simulink model "ScenarioNew"  (Simulink 7.7)
settings: Solver=ode45  StartTime=0.0  StopTime=10.0  RelTol=1e-3
undefined symbols (not defined in the file): sigbuilder_block
libraries: simulink x1
settings Model: Creator=Zsolt  LastModifiedBy=jscott
settings HardwareCC: TargetIntDivRoundTo=Zero  TargetEndianess=LittleEndian  TargetHWDeviceType=MATLAB Host  ProdEqTarget=off
settings RTWCC: SystemTargetFile=rsim.tlc  TemplateMakefile=rsim_default_tmf  Description=Rapid Simulation Target  ProcessScript=rsim_make_rtw_hook
settings RSimTargetCC: TargetFunctionLibrary=ANSI_C  ERTMultiwordTypeDef=System defined  FunctionExecutionProfile=off  CodeExecutionProfiling=off  ERTCodeCoverageTool=None  ERTMultiwordLength=256  IsPILTarget=off  EnableShiftOperators=on  PortableWordSizes=off

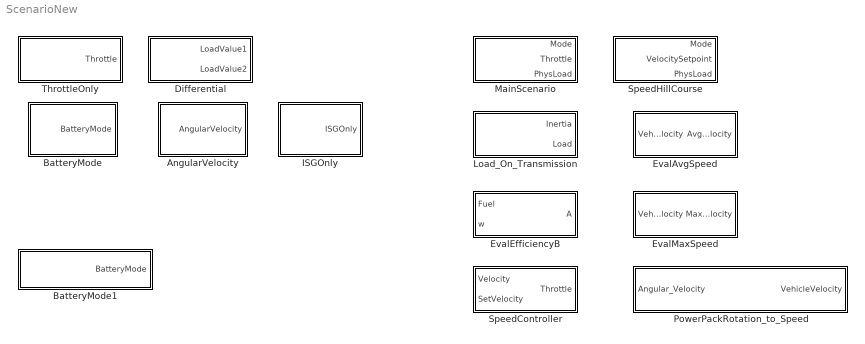
== system ScenarioNew ==
  AngularVelocity : Subsystem  Tag=STV Subsys  LoadFcn=sigbuilder_block('load');  StartFcn=sigbuilder_block('start');  StopFcn=sigbuilder_block('stop');  ClipboardFcn=sigbuilder_block('clipboard');  mask(Sigbuilder block){}
      mask help: Create and generate interchangeable groups of signals whose waveforms are piecewise linear.
      mask init:
      | if ~strcmp(get_param(bdroot(gcbh),'SimulationStatus'),'stopped') tuvar = sigbuilder_block('maskInit'); end
      settings: CopyFcn=sigbuilder_block('copy');  DeleteFcn=sigbuilder_block('delete');  ModelCloseFcn=sigbuilder_block('modelClose');  PreSaveFcn=sigbuilder_block('preSave');  NameChangeFcn=sigbuilder_block('namechange');  OpenFcn=sigbuilder_block('open',[437.25 199.5 550.5 399.75 ]);  CloseFcn=sigbuilder_block('close');
      mask Display: plot(0,0,100,100,[10,10,40,40,10],[80,20,20,80,80],[40,10],[50,50], [40,27,10],[65,72,56],[40,25,25,10],[28,28,43,43]);
  BatteryMode : Subsystem  Tag=STV Subsys  LoadFcn=sigbuilder_block('load');  StartFcn=sigbuilder_block('start');  StopFcn=sigbuilder_block('stop');  ClipboardFcn=sigbuilder_block('clipboard');  mask(Sigbuilder block){}
      mask help: Create and generate interchangeable groups of signals whose waveforms are piecewise linear.
      mask init:
      | if ~strcmp(get_param(bdroot(gcbh),'SimulationStatus'),'stopped') tuvar = sigbuilder_block('maskInit'); end
      settings: CopyFcn=sigbuilder_block('copy');  DeleteFcn=sigbuilder_block('delete');  ModelCloseFcn=sigbuilder_block('modelClose');  PreSaveFcn=sigbuilder_block('preSave');  NameChangeFcn=sigbuilder_block('namechange');  OpenFcn=sigbuilder_block('open',[437.25 199.5 550.5 399.75 ]);  CloseFcn=sigbuilder_block('close');
      mask Display: plot(0,0,100,100,[10,10,40,40,10],[80,20,20,80,80],[40,10],[50,50], [40,27,10],[65,72,56],[40,25,25,10],[28,28,43,43]);
  BatteryMode1 : Subsystem  Tag=STV Subsys  LoadFcn=sigbuilder_block('load');  StartFcn=sigbuilder_block('start');  StopFcn=sigbuilder_block('stop');  ClipboardFcn=sigbuilder_block('clipboard');  mask(Sigbuilder block){}
      mask help: Create and generate interchangeable groups of signals whose waveforms are piecewise linear.
      mask init:
      | if ~strcmp(get_param(bdroot(gcbh),'SimulationStatus'),'stopped') tuvar = sigbuilder_block('maskInit'); end
      settings: CopyFcn=sigbuilder_block('copy');  DeleteFcn=sigbuilder_block('delete');  ModelCloseFcn=sigbuilder_block('modelClose');  PreSaveFcn=sigbuilder_block('preSave');  NameChangeFcn=sigbuilder_block('namechange');  OpenFcn=sigbuilder_block('open',[437.25 199.5 550.5 399.75 ]);  CloseFcn=sigbuilder_block('close');
      mask Display: plot(0,0,100,100,[10,10,40,40,10],[80,20,20,80,80],[40,10],[50,50], [40,27,10],[65,72,56],[40,25,25,10],[28,28,43,43]);
  Differential : Subsystem
  EvalAvgSpeed : Subsystem
  EvalEfficiencyB : Subsystem
  EvalMaxSpeed : Subsystem
  ISGOnly : Subsystem  Tag=STV Subsys  LoadFcn=sigbuilder_block('load');  StartFcn=sigbuilder_block('start');  StopFcn=sigbuilder_block('stop');  ClipboardFcn=sigbuilder_block('clipboard');  mask(Sigbuilder block){}
      mask help: Create and generate interchangeable groups of signals whose waveforms are piecewise linear.
      mask init:
      | if ~strcmp(get_param(bdroot(gcbh),'SimulationStatus'),'stopped') tuvar = sigbuilder_block('maskInit'); end
      settings: CopyFcn=sigbuilder_block('copy');  DeleteFcn=sigbuilder_block('delete');  ModelCloseFcn=sigbuilder_block('modelClose');  PreSaveFcn=sigbuilder_block('preSave');  NameChangeFcn=sigbuilder_block('namechange');  OpenFcn=sigbuilder_block('open',[437.25 199.5 550.5 399.75 ]);  CloseFcn=sigbuilder_block('close');
      mask Display: plot(0,0,100,100,[10,10,40,40,10],[80,20,20,80,80],[40,10],[50,50], [40,27,10],[65,72,56],[40,25,25,10],[28,28,43,43]);
  Load_On_Transmission : Subsystem
  MainScenario : Subsystem
  PowerPackRotation_to_Speed : Subsystem
  SpeedController : Subsystem
  SpeedHillCourse : Subsystem
  ThrottleOnly : Subsystem

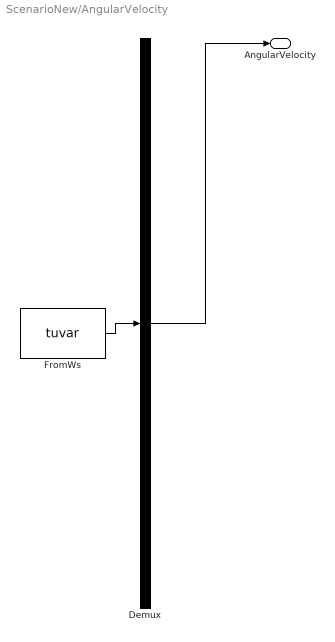
== system ScenarioNew/AngularVelocity ==
  Demux : Demux  Tag=STV Demux  Outputs=1
  FromWs : FromWorkspace  Tag=STV FromWs  VariableName=tuvar  SampleTime=0  SigBuilderData=DataTag0  VnvData=DataTag1
      SigBuilderData=|
      | common.afterFinalStr = 'Extrapolate'
      | common.sampleTime = 0
      | dataSet.timeRange = [0 100]
      | dataSet.name = 'Group 1'
      | sbobj.Groups.Name = 'Group 1'
      | sbobj.Groups.Signals.Name = 'AngularVelocity'
      | sbobj.Groups.Signals.XData = [0 50 100]
      | sbobj.Groups.Signals.YData = [0 250 0]
  AngularVelocity : Outport  Tag=STV Outport
  wires:
  FromWs/1 -> Demux/1
  Demux/1 -> AngularVelocity/1

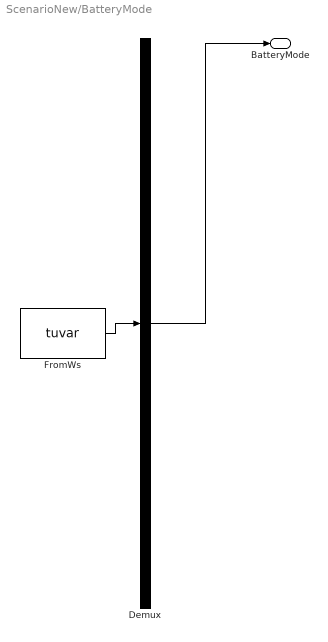
== system ScenarioNew/BatteryMode ==
  Demux : Demux  Tag=STV Demux  Outputs=1
  FromWs : FromWorkspace  Tag=STV FromWs  VariableName=tuvar  SampleTime=0  SigBuilderData=DataTag2  VnvData=DataTag3
      SigBuilderData=|
      | common.afterFinalStr = 'Extrapolate'
      | common.sampleTime = 0
      | dataSet.timeRange = [0 10000]
      | dataSet.name = 'Group 1'
      | sbobj.Groups.Name = 'Group 1'
      | sbobj.Groups.Signals.Name = 'BatteryMode'
      | sbobj.Groups.Signals.XData = [0 3.4 8.7 10.6 10.6 18.6 31.1 97 2000 2000 2400 2400 5240 5240 5580 5580 5820 5820 10000]
      | sbobj.Groups.Signals.YData = [2 2 2 2 1 1 1 1 1 2 2 1 1 0 0 2 2 0 0]
  BatteryMode : Outport  Tag=STV Outport
  wires:
  Demux/1 -> BatteryMode/1
  FromWs/1 -> Demux/1

== system ScenarioNew/BatteryMode1 ==
  Demux : Demux  Tag=STV Demux  Outputs=1
  FromWs : FromWorkspace  Tag=STV FromWs  VariableName=tuvar  SampleTime=0  SigBuilderData=DataTag4  VnvData=DataTag5
      SigBuilderData=|
      | common.afterFinalStr = 'Extrapolate'
      | common.sampleTime = 0
      | dataSet.timeRange = [0 100]
      | dataSet.name = 'Group 1'
      | sbobj.Groups.Name = 'Group 1'
      | sbobj.Groups.Signals.Name = 'BatteryMode'
      | sbobj.Groups.Signals.XData = [0 3.4 8.7 10.6 10.6 18.6 18.6 31.1 97 97 100]
      | sbobj.Groups.Signals.YData = [2 2 2 2 1 1 2 2 2 0 0]
  BatteryMode : Outport  Tag=STV Outport
  wires:
  FromWs/1 -> Demux/1
  Demux/1 -> BatteryMode/1

== system ScenarioNew/Differential ==
  Differential driver : Subsystem  Tag=STV Subsys  LoadFcn=sigbuilder_block('load');  StartFcn=sigbuilder_block('start');  StopFcn=sigbuilder_block('stop');  ClipboardFcn=sigbuilder_block('clipboard');  mask(Sigbuilder block){}
      mask help: Create and generate interchangeable groups of signals whose waveforms are piecewise linear.
      mask init:
      | if ~strcmp(get_param(bdroot(gcbh),'SimulationStatus'),'stopped') tuvar = sigbuilder_block('maskInit'); end
      settings: CopyFcn=sigbuilder_block('copy');  DeleteFcn=sigbuilder_block('delete');  ModelCloseFcn=sigbuilder_block('modelClose');  PreSaveFcn=sigbuilder_block('preSave');  NameChangeFcn=sigbuilder_block('namechange');  OpenFcn=sigbuilder_block('open',[437.25 199.5 550.5 399.75 ]);  CloseFcn=sigbuilder_block('close');
      mask Display: plot(0,0,100,100,[10,10,40,40,10],[80,20,20,80,80],[40,10],[50,50], [40,27,10],[65,72,56],[40,25,25,10],[28,28,43,43]);
  LoadValue1 : Outport
  LoadValue2 : Outport  Port=2
  wires:
  Differential driver/1(Load1) -> LoadValue1/1
  Differential driver/2(Load2) -> LoadValue2/1

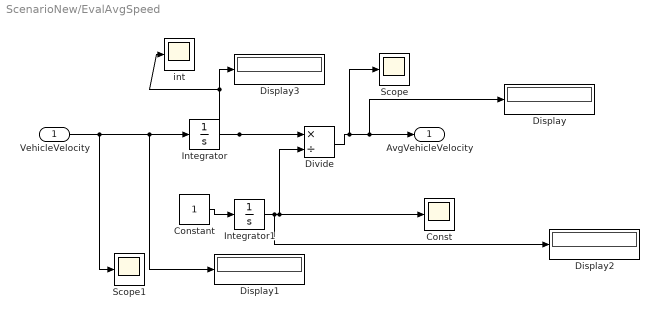
== system ScenarioNew/EvalAvgSpeed ==
  VehicleVelocity : Inport
  Const : Scope
      settings: YMin=250  YMax=4250
  Constant : Constant
  Display{,1..3} (4 alike) : Display
  Divide : Product  Inputs=*/
  Integrator : Integrator
  Integrator1 : Integrator
  Scope : Scope
      settings: YMin=250  YMax=4250  SaveName=ScopeData2
  Scope1 : Scope
      settings: YMin=250  YMax=4250  SaveName=ScopeData3
  int : Scope
      settings: YMin=250  YMax=4250  SaveName=ScopeData4
  AvgVehicleVelocity : Outport
  wires:
  Divide/1 -> Scope/1, AvgVehicleVelocity/1, Display/1
  VehicleVelocity/1 -> Scope1/1, Display1/1, Integrator/1
  Constant/1 -> Integrator1/1
  Integrator/1 -> Divide/1, Display3/1, int/1
  Integrator1/1 -> Display2/1, Divide/2, Const/1

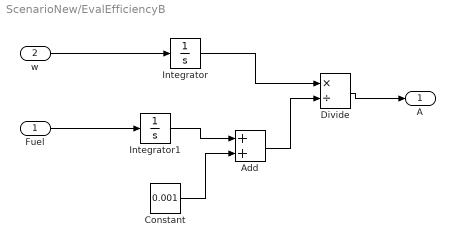
== system ScenarioNew/EvalEfficiencyB ==
  Fuel : Inport
  w : Inport  Port=2
  Add : Sum
  Constant : Constant  Value=0.001
  Divide : Product  Inputs=*/
  Integrator : Integrator
  Integrator1 : Integrator
  A : Outport
  wires:
  Divide/1 -> A/1
  Integrator1/1 -> Add/1
  Constant/1 -> Add/2
  w/1 -> Integrator/1
  Fuel/1 -> Integrator1/1
  Add/1 -> Divide/2
  Integrator/1 -> Divide/1

== system ScenarioNew/EvalMaxSpeed ==
  VehicleVelocity : Inport
  MinMax : MinMax  Function=max
  MaxVehicleVelocity : Outport
  wires:
  VehicleVelocity/1 -> MinMax/1
  MinMax/1 -> MaxVehicleVelocity/1

== system ScenarioNew/ISGOnly ==
  Demux : Demux  Tag=STV Demux  Outputs=1
  FromWs : FromWorkspace  Tag=STV FromWs  VariableName=tuvar  SampleTime=0  SigBuilderData=DataTag8  VnvData=DataTag9
      SigBuilderData=|
      | common.afterFinalStr = 'Extrapolate'
      | common.sampleTime = 0
      | dataSet.timeRange = [0 100]
      | dataSet.name = 'Group 1'
      | sbobj.Groups.Name = 'Group 1'
      | sbobj.Groups.Signals.Name = 'ISGOnly'
      | sbobj.Groups.Signals.XData = [0 8 8 30.2 30.2 37.8 37.8 66.4 66.4 77 77 100]
      | sbobj.Groups.Signals.YData = [2 2 1 1 2 2 0 0 1 1 2 2]
  ISGOnly : Outport  Tag=STV Outport
  wires:
  Demux/1 -> ISGOnly/1
  FromWs/1 -> Demux/1

== system ScenarioNew/Load_On_Transmission ==
  Differential driver : Subsystem  Tag=STV Subsys  LoadFcn=sigbuilder_block('load');  StartFcn=sigbuilder_block('start');  StopFcn=sigbuilder_block('stop');  ClipboardFcn=sigbuilder_block('clipboard');  mask(Sigbuilder block){}
      mask help: Create and generate interchangeable groups of signals whose waveforms are piecewise linear.
      mask init:
      | if ~strcmp(get_param(bdroot(gcbh),'SimulationStatus'),'stopped') tuvar = sigbuilder_block('maskInit'); end
      settings: CopyFcn=sigbuilder_block('copy');  DeleteFcn=sigbuilder_block('delete');  ModelCloseFcn=sigbuilder_block('modelClose');  PreSaveFcn=sigbuilder_block('preSave');  NameChangeFcn=sigbuilder_block('namechange');  OpenFcn=sigbuilder_block('open',[711.75 149.25 550.5 399.75 ]);  CloseFcn=sigbuilder_block('close');
      mask Display: plot(0,0,100,100,[10,10,40,40,10],[80,20,20,80,80],[40,10],[50,50], [40,27,10],[65,72,56],[40,25,25,10],[28,28,43,43]);
  Inertia : Outport
  Load : Outport  Port=2
  wires:
  Differential driver/2(Load) -> Load/1
  Differential driver/1(Inertia) -> Inertia/1

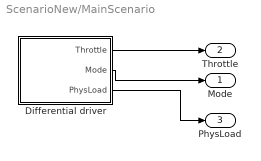
== system ScenarioNew/MainScenario ==
  Differential driver : Subsystem  Tag=STV Subsys  LoadFcn=sigbuilder_block('load');  StartFcn=sigbuilder_block('start');  StopFcn=sigbuilder_block('stop');  ClipboardFcn=sigbuilder_block('clipboard');  mask(Sigbuilder block){}
      mask help: Create and generate interchangeable groups of signals whose waveforms are piecewise linear.
      mask init:
      | if ~strcmp(get_param(bdroot(gcbh),'SimulationStatus'),'stopped') tuvar = sigbuilder_block('maskInit'); end
      settings: CopyFcn=sigbuilder_block('copy');  DeleteFcn=sigbuilder_block('delete');  ModelCloseFcn=sigbuilder_block('modelClose');  PreSaveFcn=sigbuilder_block('preSave');  NameChangeFcn=sigbuilder_block('namechange');  OpenFcn=sigbuilder_block('open',[-1510.5 -82.5 550.5 386.25 ]);  CloseFcn=sigbuilder_block('close');
      mask Display: plot(0,0,100,100,[10,10,40,40,10],[80,20,20,80,80],[40,10],[50,50], [40,27,10],[65,72,56],[40,25,25,10],[28,28,43,43]);
  Mode : Outport
  Throttle : Outport  Port=2
  PhysLoad : Outport  Port=3
  wires:
  Differential driver/1(Throttle) -> Throttle/1
  Differential driver/2(Mode) -> Mode/1
  Differential driver/3(PhysLoad) -> PhysLoad/1

== system ScenarioNew/PowerPackRotation_to_Speed ==
  Angular_Velocity : Inport
  Gain : Gain  Gain=11.3
  VehicleVelocity : Outport
  wires:
  Gain/1 -> VehicleVelocity/1
  Angular_Velocity/1 -> Gain/1

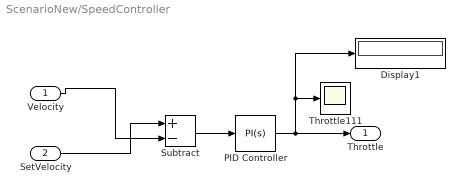
== system ScenarioNew/SpeedController ==
  Velocity : Inport
  SetVelocity : Inport  Port=2
  Display1 : Display
  PID Controller : simulink/Continuous/PID Controller  SystemSampleTime=-1  Controller=PI  TimeDomain=Continuous-time  SampleTime=1  IntegratorMethod=Forward Euler  FilterMethod=Forward Euler  Form=Parallel  P=0.01  I=0.1  D=0  N=100  InitialConditionSource=internal  InitialConditionForIntegrator=0  InitialConditionForFilter=0  ExternalReset=none  LimitOutput=on  UpperSaturationLimit=1  LowerSaturationLimit=0  LinearizeAsGain=off  AntiWindupMode=clamping  Kb=1  TrackingMode=off  Kt=1  PParamMin=[]  PParamMax=[]  IParamMin=[]  IParamMax=[]  DParamMin=[]  DParamMax=[]  NParamMin=[]  NParamMax=[]  KbParamMin=[]  KbParamMax=[]  KtParamMin=[]  KtParamMax=[]  POutMin=[]  POutMax=[]  IOutMin=[]  IOutMax=[]  DOutMin=[]  DOutMax=[]  NOutMin=[]  NOutMax=[]  KbOutMin=[]  KbOutMax=[]  KtOutMin=[]  KtOutMax=[]  IntegratorOutMin=[]  IntegratorOutMax=[]  FilterOutMin=[]  FilterOutMax=[]  SumOutMin=[]  SumOutMax=[]  SumI1OutMin=[]  SumI1OutMax=[]  SumI2OutMin=[]  SumI2OutMax=[]  SumI3OutMin=[]  SumI3OutMax=[]  SumDOutMin=[]  SumDOutMax=[]  SaturationOutMin=[]  SaturationOutMax=[]  IntegratorContinuousStateAttributes=''  IntegratorStateMustResolveToSignalObject=off  IntegratorRTWStateStorageClass=Auto  FilterContinuousStateAttributes=''  FilterStateMustResolveToSignalObject=off  FilterRTWStateStorageClass=Auto
  Subtract : Sum  Inputs=+-
  Throttle111 : Scope
      settings: TimeRange=100  YMin=-3  YMax=8
  Throttle : Outport
  wires:
  Velocity/1 -> Subtract/2
  SetVelocity/1 -> Subtract/1
  Subtract/1 -> PID Controller/1
  PID Controller/1 -> Throttle/1, Throttle111/1, Display1/1

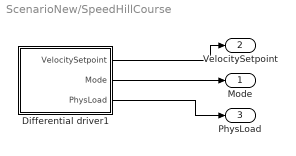
== system ScenarioNew/SpeedHillCourse ==
  Differential driver1 : Subsystem  Tag=STV Subsys  LoadFcn=sigbuilder_block('load',[-1325.25 309.75 969.75 501.75 ]);  StartFcn=sigbuilder_block('start');  StopFcn=sigbuilder_block('stop');  ClipboardFcn=sigbuilder_block('clipboard');  mask(Sigbuilder block){}
      mask help: Create and generate interchangeable groups of signals whose waveforms are piecewise linear.
      mask init:
      | if ~strcmp(get_param(bdroot(gcbh),'SimulationStatus'),'stopped') tuvar = sigbuilder_block('maskInit'); end
      settings: CopyFcn=sigbuilder_block('copy');  DeleteFcn=sigbuilder_block('delete');  ModelCloseFcn=sigbuilder_block('modelClose');  PreSaveFcn=sigbuilder_block('preSave');  NameChangeFcn=sigbuilder_block('namechange');  OpenFcn=sigbuilder_block('open',[165 24 969.75 501.75 ]);  CloseFcn=sigbuilder_block('close');
      mask Display: plot(0,0,100,100,[10,10,40,40,10],[80,20,20,80,80],[40,10],[50,50], [40,27,10],[65,72,56],[40,25,25,10],[28,28,43,43]);
  Mode : Outport
  VelocitySetpoint : Outport  Port=2
  PhysLoad : Outport  Port=3
  wires:
  Differential driver1/1(VelocitySetpoint) -> VelocitySetpoint/1
  Differential driver1/2(Mode) -> Mode/1
  Differential driver1/3(PhysLoad) -> PhysLoad/1

== system ScenarioNew/ThrottleOnly ==
  Throttle signal : Subsystem  Tag=STV Subsys  LoadFcn=sigbuilder_block('load');  StartFcn=sigbuilder_block('start');  StopFcn=sigbuilder_block('stop');  ClipboardFcn=sigbuilder_block('clipboard');  mask(Sigbuilder block){}
      mask help: Create and generate interchangeable groups of signals whose waveforms are piecewise linear.
      mask init:
      | if ~strcmp(get_param(bdroot(gcbh),'SimulationStatus'),'stopped') tuvar = sigbuilder_block('maskInit'); end
      settings: CopyFcn=sigbuilder_block('copy');  DeleteFcn=sigbuilder_block('delete');  ModelCloseFcn=sigbuilder_block('modelClose');  PreSaveFcn=sigbuilder_block('preSave');  NameChangeFcn=sigbuilder_block('namechange');  OpenFcn=sigbuilder_block('open',[437.25 199.5 550.5 399.75 ]);  CloseFcn=sigbuilder_block('close');
      mask Display: plot(0,0,100,100,[10,10,40,40,10],[80,20,20,80,80],[40,10],[50,50], [40,27,10],[65,72,56],[40,25,25,10],[28,28,43,43]);
  Throttle : Outport
  wires:
  Throttle signal/1(Throttle) -> Throttle/1

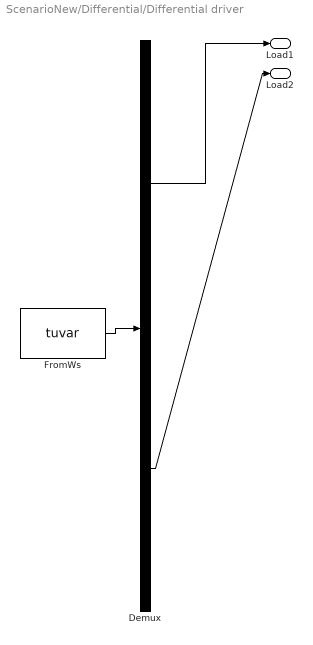
== system ScenarioNew/Differential/Differential driver ==
  Demux : Demux  Tag=STV Demux  Outputs=2
  FromWs : FromWorkspace  Tag=STV FromWs  VariableName=tuvar  SampleTime=0  SigBuilderData=DataTag6  VnvData=DataTag7
      SigBuilderData=|
      | common.afterFinalStr = 'Extrapolate'
      | common.sampleTime = 0
      | dataSet.timeRange = [0 100]
      | dataSet.name = 'Group 1'
      | sbobj.Groups.Name = 'Group 1'
      | sbobj.Groups.Signals(1).Name = 'Load1'
      | sbobj.Groups.Signals(1).XData = [0 4 4 7 20 20.8 36.8 38 67.8 70 100]
      | sbobj.Groups.Signals(1).YData = [0.03 0.03 0.025 1 1 0.595 0.595 1 1 0.02 0.02]
      | sbobj.Groups.Signals(2).Name = 'Load2'
      | sbobj.Groups.Signals(2).XData = [0 40 40 60 60 100]
      | sbobj.Groups.Signals(2).YData = [0 0 1 1 0 0]
  Load1 : Outport  Tag=STV Outport
  Load2 : Outport  Tag=STV Outport  Port=2
  wires:
  Demux/1 -> Load1/1
  FromWs/1 -> Demux/1
  Demux/2 -> Load2/1

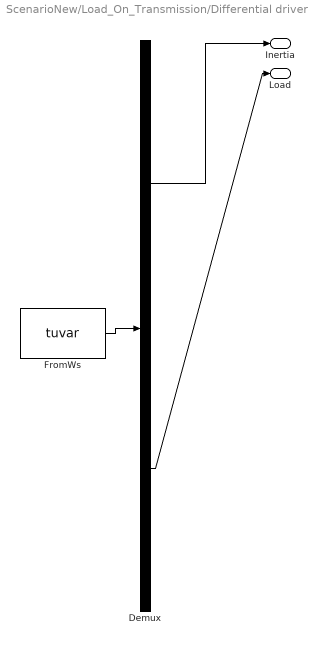
== system ScenarioNew/Load_On_Transmission/Differential driver ==
  Demux : Demux  Tag=STV Demux  Outputs=2
  FromWs : FromWorkspace  Tag=STV FromWs  VariableName=tuvar  SampleTime=0  SigBuilderData=DataTag10  VnvData=DataTag11
      SigBuilderData=|
      | common.afterFinalStr = 'Extrapolate'
      | common.sampleTime = 0
      | dataSet.timeRange = [0 100]
      | dataSet.name = 'Group 1'
      | sbobj.Groups.Name = 'Group 1'
      | sbobj.Groups.Signals(1).Name = 'Inertia'
      | sbobj.Groups.Signals(1).XData = [0 4 4 7 7 20 20 20.8 36.8 100]
      | sbobj.Groups.Signals(1).YData = [50 50 44.5 45.5 47 47 47 46.5 46.5 46.5]
      | sbobj.Groups.Signals(2).Name = 'Load'
      | sbobj.Groups.Signals(2).XData = [0 40 60 100]
      | sbobj.Groups.Signals(2).YData = [10 10 10 10]
  Inertia : Outport  Tag=STV Outport
  Load : Outport  Tag=STV Outport  Port=2
  wires:
  Demux/1 -> Inertia/1
  FromWs/1 -> Demux/1
  Demux/2 -> Load/1

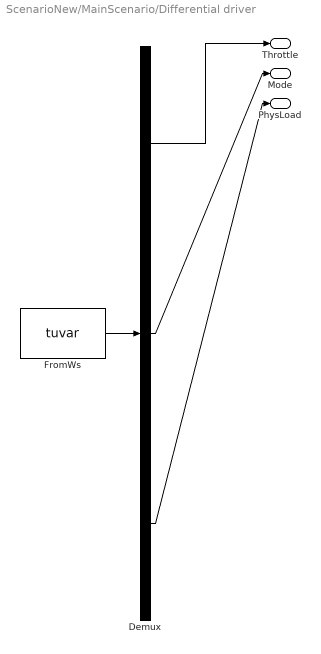
== system ScenarioNew/MainScenario/Differential driver ==
  Demux : Demux  Tag=STV Demux  Outputs=3
  FromWs : FromWorkspace  Tag=STV FromWs  VariableName=tuvar  SampleTime=0  SigBuilderData=DataTag12  VnvData=DataTag13
      SigBuilderData=|
      | common.afterFinalStr = 'Extrapolate'
      | common.sampleTime = 0
      | dataSet.timeRange = [0 100]
      | dataSet.name = 'Group 1'
      | sbobj.Groups.Name = 'Group 1'
      | sbobj.Groups.Signals(1).Name = 'Throttle'
      | sbobj.Groups.Signals(1).XData = [0 4 4 7 20 20.8 36.8 38 67.8 70 100]
      | sbobj.Groups.Signals(1).YData = [0.03 0.03 0.025 1 1 0.595 0.595 1 1 0.02 0.02]
      | sbobj.Groups.Signals(2).Name = 'Mode'
      | sbobj.Groups.Signals(2).XData = [0 40 60 100]
      | sbobj.Groups.Signals(2).YData = [0 0 0 0]
      | sbobj.Groups.Signals(3).Name = 'PhysLoad'
      | sbobj.Groups.Signals(3).XData = [0 40 60 100]
      | sbobj.Groups.Signals(3).YData = [10 10 10 10]
  Throttle : Outport  Tag=STV Outport
  Mode : Outport  Tag=STV Outport  Port=2
  PhysLoad : Outport  Tag=STV Outport  Port=3
  wires:
  Demux/2 -> Mode/1
  FromWs/1 -> Demux/1
  Demux/1 -> Throttle/1
  Demux/3 -> PhysLoad/1

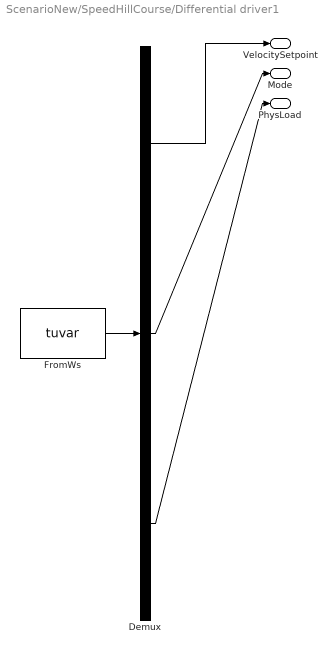
== system ScenarioNew/SpeedHillCourse/Differential driver1 ==
  Demux : Demux  Tag=STV Demux  Outputs=3
  FromWs : FromWorkspace  Tag=STV FromWs  VariableName=tuvar  SampleTime=0  SigBuilderData=DataTag14  VnvData=DataTag15
      SigBuilderData=|
      | common.afterFinalStr = 'Extrapolate'
      | common.sampleTime = 0
      | dataSet.timeRange = [0 100]
      | dataSet.name = 'Group 1'
      | sbobj.Groups.Name = 'Group 1'
      | sbobj.Groups.Signals(1).Name = 'VelocitySetpoint'
      | sbobj.Groups.Signals(1).XData = [0 4 36.8 67.8 70 100]
      | sbobj.Groups.Signals(1).YData = [16800 13300 12000 11200 11200 10800]
      | sbobj.Groups.Signals(2).Name = 'Mode'
      | sbobj.Groups.Signals(2).XData = [0 40 40 60 60 100]
      | sbobj.Groups.Signals(2).YData = [0 0 1 1 0 0]
      | sbobj.Groups.Signals(3).Name = 'PhysLoad'
      | sbobj.Groups.Signals(3).XData = [0 40 60 100]
      | sbobj.Groups.Signals(3).YData = [10 10 10 10]
  VelocitySetpoint : Outport  Tag=STV Outport
  Mode : Outport  Tag=STV Outport  Port=2
  PhysLoad : Outport  Tag=STV Outport  Port=3
  wires:
  Demux/3 -> PhysLoad/1
  Demux/1 -> VelocitySetpoint/1
  FromWs/1 -> Demux/1
  Demux/2 -> Mode/1

== system ScenarioNew/ThrottleOnly/Throttle signal ==
  Demux : Demux  Tag=STV Demux  Outputs=1
  FromWs : FromWorkspace  Tag=STV FromWs  VariableName=tuvar  SampleTime=0  SigBuilderData=DataTag16  VnvData=DataTag17
      SigBuilderData=|
      | common.afterFinalStr = 'Extrapolate'
      | common.sampleTime = 0
      | dataSet.timeRange = [0 100]
      | dataSet.name = 'Group 1'
      | sbobj.Groups.Name = 'Group 1'
      | sbobj.Groups.Signals.Name = 'Throttle'
      | sbobj.Groups.Signals.XData = [0 4 4 7 20 20.8 36.8 38 67.8 70 100]
      | sbobj.Groups.Signals.YData = [0.03 0.03 0.025 1 1 0.595 0.595 1 1 0.02 0.02]
  Throttle : Outport  Tag=STV Outport
  wires:
  FromWs/1 -> Demux/1
  Demux/1 -> Throttle/1
